simulink model "Modello_attuatore"  (R2023a)
settings: Solver=ode14x  StartTime=0.0  StopTime=3  FixedStep=dt_sim  RelTol=1e-3
values from neighbouring files (symbols this model uses):
  A1_la = 5.710000e-003    (= 0.00571)    [C1_Actuator_1_Data.m]
  A2_la = 5.710000e-003    (= 0.00571)    [C1_Actuator_1_Data.m]
  a_jetpipe_area = 0    [B2_Main_file_Double_Active_Standby_System.m]
  A_svfb = 79.12.*1E-9.*sqrt(pi)    [B2_Main_file_Double_Active_Standby_System.m]
  a_svfb0_1 = 1E-3    (= 0.001)    [B2_Main_file_Double_Active_Standby_System.m]
  a_svfb0_2 = 0    [B2_Main_file_Double_Active_Standby_System.m]
  Afl_sv = dfl_sv^2*pi/4    (= 2.01519637574e-09)    [C1_Actuator_1_Data.m]
  Ag_sv = 18e-6    (= 1.8e-05)    [C1_Actuator_1_Data.m]
  air_gap0_1 = 0    [B2_Main_file_Double_Active_Standby_System.m]
  air_gap_fault_time = 10000    [B2_Main_file_Double_Active_Standby_System.m]
  Asp_sv = 1.35e-5    (= 1.35e-05)    [C1_Actuator_1_Data.m]
  B0_sv = 0.460    (= 0.46)    [C1_Actuator_1_Data.m]
  b_airgap = 0.3    [B2_Main_file_Double_Active_Standby_System.m]
  b_fbspring = 2E-3    (= 0.002)    [B2_Main_file_Double_Active_Standby_System.m]
  b_max = 0*0.0001    (= 0)    [C1_Actuator_1_Data.m]
  beta = 800000000    [D4_Fluid.m]    (also in Rapporto_di_trasmissione.m = acos((L-t.*cos(alpha))./s))
  beta_LVDT = 0    [aggiunte.m]
  bf_sv = 0.45    [C1_Actuator_1_Data.m]
  bsp_sv = 0.25    [C1_Actuator_1_Data.m]
  C_svfb = 1    [B2_Main_file_Double_Active_Standby_System.m]
  Cdmax_sv = 0.7392    [C1_Actuator_1_Data.m]
  Cdmin_sv = 0.6428    [C1_Actuator_1_Data.m]
  CLa = 900000    [aggiunte.m]
  Csa_la = 0.02*sqrt(Ksa_la*Meq_la)    [C1_Actuator_1_Data.m]
  Del_on = 1    [B2_Main_file_Double_Active_Standby_System.m]
  demag0_1 = 0    [B2_Main_file_Double_Active_Standby_System.m]
  dfl_sv = 5.0654e-5    (= 5.0654e-05)    [C1_Actuator_1_Data.m]
  dt_sim = 1e-5    (= 1e-05)    [B2_Main_file_Double_Active_Standby_System.m]
  enable_jetpipe_distorsion = 0    [B2_Main_file_Double_Active_Standby_System.m]
  F_att_sv = 4    [C1_Actuator_1_Data.m]
  FH = FH+0.175*pi*Dd_se(ii)*(-0.884+0.0206*Hs_se(ii)-0.0001*(Hs_se(ii))^2)*Tw_se(ii)    [D2_Data_seal.m]
  first_cycle = 0    [B2_Main_file_Double_Active_Standby_System.m]
  flight_hours = 8    [B2_Main_file_Double_Active_Standby_System.m]
  g_sv = G_sv/l0_sv    (= 0)    [C1_Actuator_1_Data.m]
  Gamma_la = 1.667e4    (= 16670)    [C1_Actuator_1_Data.m]
  gap_ms = 0    [C1_Actuator_1_Data.m]
  Gq_sv = 0.069    [C1_Actuator_1_Data.m]
  Gust_stiffness_jetpipe = 1e8    (= 100000000)    [B2_Main_file_Double_Active_Standby_System.m]
  Gust_threshold = 10000    [B2_Main_file_Double_Active_Standby_System.m]
  h_fbspring = 1E-3    (= 0.001)    [B2_Main_file_Double_Active_Standby_System.m]
  h_sv = H_sv/l0_sv    (= 0)    [C1_Actuator_1_Data.m]
  hr_sv = 6e-6    (= 6e-06)    [C1_Actuator_1_Data.m]
  hyd_fluid_repl = 20    [B2_Main_file_Double_Active_Standby_System.m]
  imax_sv = 8e-3    (= 0.008)    [C1_Actuator_1_Data.m]
  Ja_sv = 1.0575e-5    (= 1.0575e-05)    [C1_Actuator_1_Data.m]
  jetpipe_initialpos = 0    [B2_Main_file_Double_Active_Standby_System.m]
  jetpipe_passage_area = 1    [B2_Main_file_Double_Active_Standby_System.m]
  k_airgap = 0.5/100*0.01    (= 5e-05)    [B2_Main_file_Double_Active_Standby_System.m]
  k_c0_jetpipe_area = 0*1e-1    (= 0)    [B2_Main_file_Double_Active_Standby_System.m]
  k_sv = mup_sv*Vp_sv/(2*B0_sv*l0_sv)-1    (= 16.0383594613)    [C1_Actuator_1_Data.m]
  Kf_sv = 301.6    [C1_Actuator_1_Data.m]
  KFPi = zeros(m,1)    [D2_Data_seal.m]
  Kli1 = 0    [C1_Actuator_1_Data.m]
  Kli2 = 0    [C1_Actuator_1_Data.m]
  Ksa_la = 12480000    [C1_Actuator_1_Data.m]
  Kw_sv = 14.5    [C1_Actuator_1_Data.m]
  l0_sv = 0.5e-3    (= 0.0005)    [C1_Actuator_1_Data.m]
  L_c = imax_sv    (= 0.008)    [C1_Actuator_1_Data.m]
  L_la1 = 0.059900    (= 0.0599)    [C1_Actuator_1_Data.m]
  L_la2 = 0.084800    (= 0.0848)    [C1_Actuator_1_Data.m]
  la_sv = 41e-3    (= 0.041)    [C1_Actuator_1_Data.m]
  lambda_LVDT = 0*0.005*1.5    (= 0)    [aggiunte.m]
  lf = 0.025    [C1_Actuator_1_Data.m]    (also in C2_Actuator_2_Data.m)
  LVDTsize0 = 1    [aggiunte.m]
  m_thermal = 0    [B2_Main_file_Double_Active_Standby_System.m]
  Mcyl_la = 30.425550    (= 30.42555)    [C1_Actuator_1_Data.m]
  Mrod_la = 11.313490    (= 11.31349)    [C1_Actuator_1_Data.m]
  msp_sv = 0.005    [C1_Actuator_1_Data.m]
  mua_sv = 4*pi/1e7    (= 1.25663706144e-06)    [C1_Actuator_1_Data.m]
  mup_sv = 1.1*4*pi/1e7    (= 1.38230076758e-06)    [C1_Actuator_1_Data.m]
  n1_sv = 1140    [C1_Actuator_1_Data.m]
  n2_sv = 1140    [C1_Actuator_1_Data.m]
  n_svfb = 3    [B2_Main_file_Double_Active_Standby_System.m]
  null_shift = -1+2*rand(1,1)    [B2_Main_file_Double_Active_Standby_System.m]
  null_shift_sign = -1+((-1+2*rand(1,1))>=0)*2    [B2_Main_file_Double_Active_Standby_System.m]
  OV_R1 = 0*2.344e-05    (= 0)    [C1_Actuator_1_Data.m]
  OV_R2 = 0*2.344e-05    (= 0)    [C1_Actuator_1_Data.m]
  OV_S1 = 0*2.344e-05    (= 0)    [C1_Actuator_1_Data.m]
  OV_S2 = 0*2.344e-05    (= 0)    [C1_Actuator_1_Data.m]
  P01_la = Pmean-DP_eq    [C1_Actuator_1_Data.m]
  P02_la = Pmean+DP_eq    [C1_Actuator_1_Data.m]
  perc_passage_area0_1 = 0    [B2_Main_file_Double_Active_Standby_System.m]
  Pocl_A = 0    [C1_Actuator_1_Data.m]
  Pocl_B = 0    [C1_Actuator_1_Data.m]
  Pr = 600000    [B2_Main_file_Double_Active_Standby_System.m]
  Ps = 35000000    [B2_Main_file_Double_Active_Standby_System.m]
  R_th1 = 0    [B2_Main_file_Double_Active_Standby_System.m]
  Remax_sv = 5000    [C1_Actuator_1_Data.m]
  Resistance = 1    [C1_Actuator_1_Data.m]
  rj_sv = 1e-6    (= 1e-06)    [C1_Actuator_1_Data.m]
  Rp02_svspring = 1014    [B2_Main_file_Double_Active_Standby_System.m]
  sigma_0LVDT = 0*0.01*1.5*5    (= 0)    [aggiunte.m]
  ST_AD = ceil(10000/fs_AD)/10000    [C1_Actuator_1_Data.m]
  sv_crackON1 = 0    [B2_Main_file_Double_Active_Standby_System.m]
  sv_crackON2 = 0    [B2_Main_file_Double_Active_Standby_System.m]
  T0 = 0    [aggiunte.m]
  tau_w1 = 0    [B2_Main_file_Double_Active_Standby_System.m]
  Temperature_threshold = 0    [B2_Main_file_Double_Active_Standby_System.m]
  V01_la = (Vm_la1+A1_la*(L_la1+x0_la))    (= 0.00040017393)    [C1_Actuator_1_Data.m]
  V02_la = (Vm_la2+A2_la*(L_la2-x0_la))    (= 0.00056652336)    [C1_Actuator_1_Data.m]
  Voltage_com = Resistance    (= 1)    [C1_Actuator_1_Data.m]
  Vp_sv = 5.67e3    (= 5670)    [C1_Actuator_1_Data.m]
  w_fb = 310    [C1_Actuator_1_Data.m]
  w_sv = W_sv/l0_sv    (= 0)    [C1_Actuator_1_Data.m]
  wsp_sv = 0.009334348785340    (= 0.00933434878534)    [C1_Actuator_1_Data.m]
  x0_la = 0    [C1_Actuator_1_Data.m]
  xf_sv_max = 3.05e-5    (= 3.05e-05)    [C1_Actuator_1_Data.m]
  xmax_sb = 5.5e-3    (= 0.0055)    [C1_Actuator_1_Data.m]
  xspmax_sv = 0.001250    (= 0.00125)    [C1_Actuator_1_Data.m]
  z_fb = 0.5    [C1_Actuator_1_Data.m]
undefined symbols (not defined in the file or in its folder): magnitude, Newton, R_sp_C, Raphson
libraries: simulink x13
(part 1 of 3)
settings Model: SimulationMode=accelerator  Creator=ciro1  LastModifiedBy=ciro1

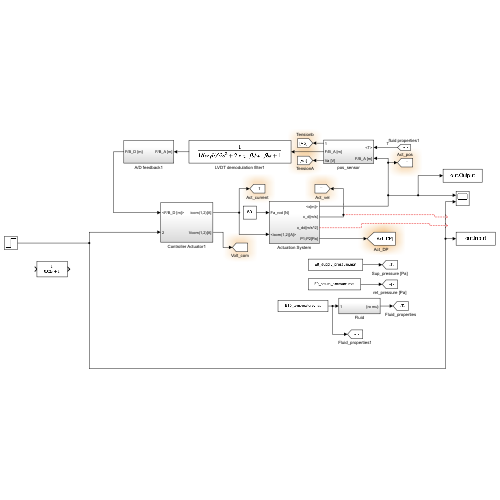
[thumbnail: Simulink's stored preview of the top-level diagram]
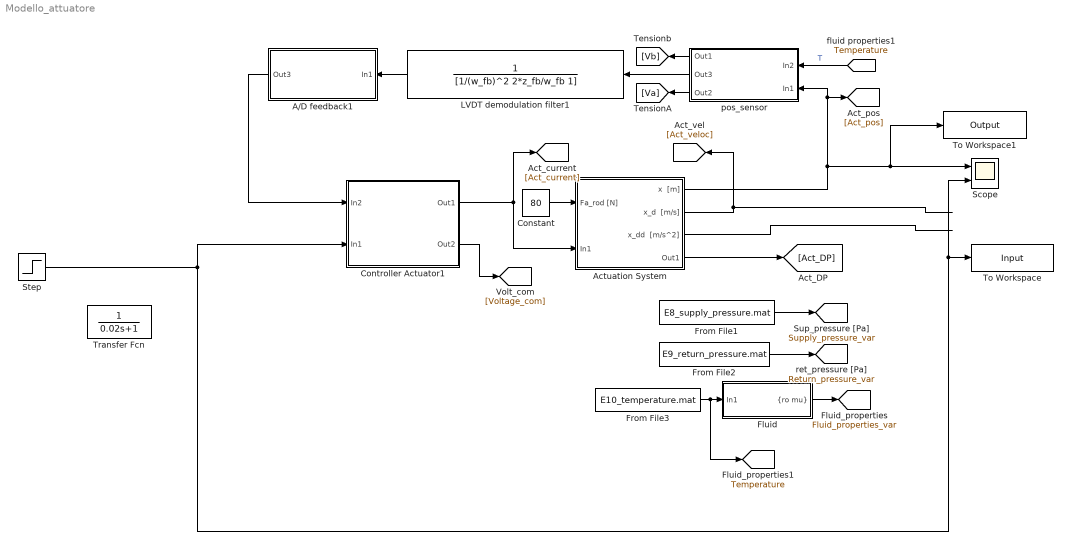
== system Modello_attuatore ==
  A/D feedback1 : Subsystem
  Actuation System : Subsystem
  Constant : Constant  Value=80
  Controller Actuator1 : Subsystem
  Fluid : Subsystem
  From File1 : FromFile  FileName=E8_supply_pressure.mat  SampleTime=dt_sim
  From File2 : FromFile  FileName=E9_return_pressure.mat  SampleTime=dt_sim
  From File3 : FromFile  FileName=E10_temperature.mat  SampleTime=dt_sim
  LVDT demodulation filter1 : TransferFcn  Denominator=[1/(w_fb)^2 2*z_fb/w_fb 1]
  Scope : Scope  NumInputPorts=2
  Step : Step  Time=0.1  After=0.02  SampleTime=0
  To Workspace : ToWorkspace  VariableName=Input  SampleTime=-1
  To Workspace1 : ToWorkspace  VariableName=Output  SampleTime=-1
  Transfer Fcn : TransferFcn  Denominator=[0.02 1]
  pos_sensor : Subsystem
  tag scope: Fluid_properties_var=global, Return_pressure_var=global, Supply_pressure_var=global, Temperature=global
  wires:
  pos_sensor/1(Out1) -> [Vb]
  pos_sensor/2(Out3) -> LVDT demodulation filter1/1
  A/D feedback1/1(Out3) -> Controller Actuator1/1(In2)
  Actuation System/3(x_dd  [m/s^2]) -> ?
  [Temperature] -> pos_sensor/1(In2)  "T"
  pos_sensor/3(Out2) -> [Va]
  Actuation System/2(x_d  [m/s]) -> [Act_veloc]
  Actuation System/4(Out1) -> [Act_DP]
  LVDT demodulation filter1/1 -> A/D feedback1/1(In1)
  Actuation System/1(x  [m]) -> To Workspace1/1, Scope/1, pos_sensor/2(In1), [Act_pos]
  Controller Actuator1/1(Out1) -> [Act_current], Actuation System/2(In1)
  Controller Actuator1/2(Out2) -> [Voltage_com]
  Fluid/1("{ro mu}") -> [Fluid_properties_var]
  From File2/1 -> [Return_pressure_var]
  From File3/1 -> [Temperature], Fluid/1(In1)
  From File1/1 -> [Supply_pressure_var]
  Step/1 -> Controller Actuator1/2(In1), Scope/2, To Workspace/1
  Constant/1 -> Actuation System/1(Fa_rod [N])

== system Modello_attuatore/A//D feedback1 ==
  In1 : Inport
  L_hight[ft]2 : Constant  Value=Del_on
  Product : Product  RndMeth=Zero
  Quantizer : Quantizer  QuantizationInterval=QI_AD
  Quantizer1 : Quantizer  QuantizationInterval=QI_AD
  "Sampler " : ZeroOrderHold  SampleTime=ST_AD
  Sum : Sum  Inputs=|++
  Uniform Random Number1 : UniformRandomNumber  Minimum=-4*2.5757e-006  Maximum=4*2.5757e-006  SampleTime=1
  Out3 : Outport
  wires:
  "Sampler "/1 -> Quantizer/1
  In1/1 -> "Sampler "/1  "F/B_A [m]"
  Uniform Random Number1/1 -> Quantizer1/1
  Quantizer/1 -> Sum/1  "F/B_D [m]"
  Sum/1 -> Out3/1  "F/B_D [m]"
  Product/1 -> Sum/2
  Quantizer1/1 -> Product/1  "Noise A/D"
  L_hight[ft]2/1 -> Product/2

== system Modello_attuatore/Actuation System ==
  Fa_rod [N] : Inport
  In1 : Inport  Port=2
  A2[m2]1 : Gain  Gain=60000
  Actuator : Subsystem
  Mux1 : Mux  Inputs=2
  Scope : Scope
  Servovalve : Subsystem
  imposed shutoff valve external position : Constant  Value=xmax_sb
  x  [m] : Outport
  x_d  [m/s] : Outport  Port=2
  x_dd  [m/s^2] : Outport  Port=3
  Out1 : Outport  Port=4
  wires:
  In1/1 -> Servovalve/2(In1)
  Actuator/2(Out3) -> x  [m]/1
  Actuator/3(Out1) -> x_d  [m/s]/1  "x_d[m/s]"
  Servovalve/1(Out4) -> Mux1/1, Actuator/1(In1)
  Servovalve/2(Out1) -> Actuator/2(In3), Mux1/2
  Actuator/1(Out2) -> Out1/1, Servovalve/1(In2)  "P1;P2[Pa]"
  imposed shutoff valve external position/1 -> Servovalve/3(In3)  "X_shutoff [m]"
  Mux1/1 -> A2[m2]1/1
  A2[m2]1/1 -> Scope/1
  Fa_rod [N]/1 -> Actuator/3(" ")
  Actuator/4(Out5) -> x_dd  [m/s^2]/1  "x_dd[m/s^2]"

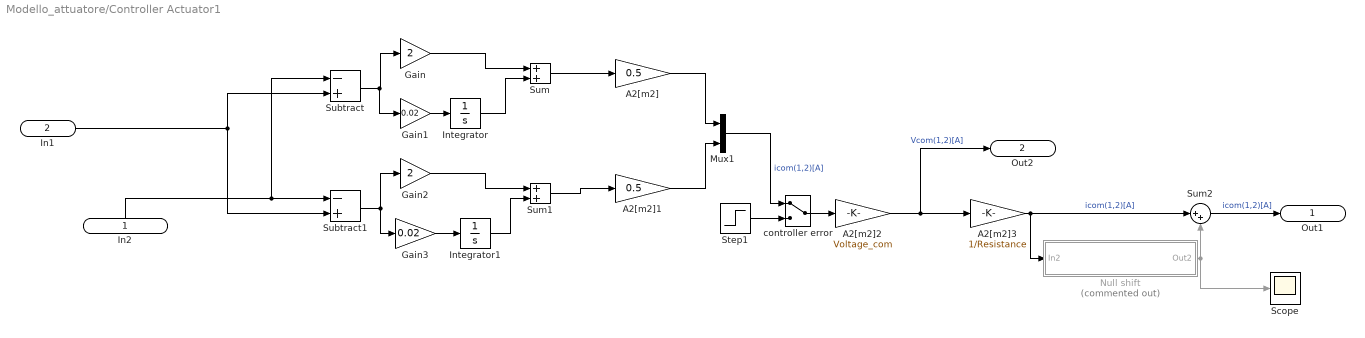
== system Modello_attuatore/Controller Actuator1 ==
  In2 : Inport
  In1 : Inport  Port=2
  A2[m2] : Gain  Gain=0.5
  A2[m2]1 : Gain  Gain=0.5
  A2[m2]2 : Gain  Gain=Voltage_com
  A2[m2]3 : Gain  Gain=1/Resistance
  Gain : Gain  Gain=2
  Gain1 : Gain  Gain=0.02
  Gain2 : Gain  Gain=2
  Gain3 : Gain  Gain=0.02
  Integrator : Integrator
  Integrator1 : Integrator
  Mux1 : Mux  Inputs=2
  Null shift : Subsystem  Commented=on
  Scope : Scope
  Step1 : Step  Time=0.3  After=L_c  SampleTime=0
  Subtract : Sum  Inputs=-+
  Subtract1 : Sum  Inputs=-+
  Sum : Sum
  Sum1 : Sum
  Sum2 : Sum  Inputs=|++
  controller error : ManualSwitch
  Out1 : Outport
  Out2 : Outport  Port=2
  wires:
  A2[m2]1/1 -> Mux1/2
  A2[m2]/1 -> Mux1/1
  In1/1 -> Subtract1/2, Subtract/2
  Mux1/1 -> controller error/1  "icom(1,2)[A]"
  controller error/1 -> A2[m2]2/1
  Step1/1 -> controller error/2
  A2[m2]2/1 -> A2[m2]3/1, Out2/1  "Vcom(1,2)[A]"
  A2[m2]3/1 -> Sum2/1, Null shift/1(In2)  "icom(1,2)[A]"
  Null shift/1(Out2) -> Sum2/2, Scope/1
  Sum2/1 -> Out1/1  "icom(1,2)[A]"
  Gain/1 -> Sum/1
  Subtract/1 -> Gain1/1, Gain/1
  Subtract1/1 -> Gain3/1, Gain2/1
  Gain2/1 -> Sum1/1
  Sum1/1 -> A2[m2]1/1
  Sum/1 -> A2[m2]/1
  In2/1 -> Subtract/1, Subtract1/1
  Gain1/1 -> Integrator/1
  Integrator/1 -> Sum/2
  Gain3/1 -> Integrator1/1
  Integrator1/1 -> Sum1/2

== system Modello_attuatore/Fluid ==
  In1 : Inport
  Mux2 : Mux  Inputs=2
  Product2 : Product  RndMeth=Zero
  tt : Fcn  Expr=(-0.85*u(1)+1015.4)*(1+20/8000)
  tt1 : Fcn  Expr=(1e-6*10^(0.3829*log10(u(1) +51)^4-1.8481*log10(u(1) +51)^3+2.2079*log10(u(1) +51)^2-1.1052*log10(u(1) +51)+2.9544))
  "{ro mu}" : Outport
  tag scope: only_viscosity_var=global
  wires:
  In1/1 -> tt1/1, tt/1
  tt/1 -> Mux2/1, Product2/1  "ro"
  Product2/1 -> Mux2/2, [only_viscosity_var]  "mu"
  tt1/1 -> Product2/2
  Mux2/1 -> "{ro mu}"/1

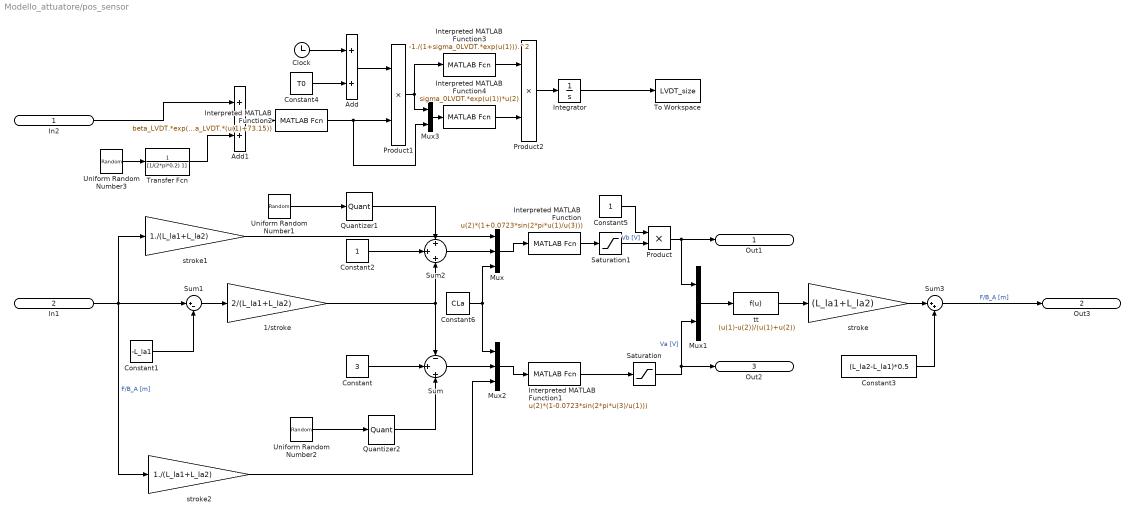
== system Modello_attuatore/pos_sensor ==
  In2 : Inport
  In1 : Inport  Port=2
  1/stroke : Gain  Gain=2/(L_la1+L_la2)  SaturateOnIntegerOverflow=on  OutDataTypeStr=Inherit: Same as input  ParamDataTypeStr=Inherit: Same as input
  Add : Sum
  Add1 : Sum
  Clock : Clock
  Constant : Constant  Value=3
  Constant1 : Constant  Value=-L_la1
  Constant2 : Constant
  Constant3 : Constant  Value=(L_la2-L_la1)*0.5
  Constant4 : Constant  Value=T0
  Constant5 : Constant
  Constant6 : Constant  Value=CLa
  Integrator : Integrator  InitialCondition=LVDTsize0
  Interpreted MATLAB Function : MATLABFcn  MATLABFcn=u(2)*(1+0.0723*sin(2*pi*u(1)/u(3)))
  Interpreted MATLAB Function1 : MATLABFcn  MATLABFcn=u(2)*(1-0.0723*sin(2*pi*u(3)/u(1)))
  Interpreted MATLAB Function2 : MATLABFcn  MATLABFcn=beta_LVDT.*exp(lambda_LVDT.*(u(1)+73.15))
  Interpreted MATLAB Function3 : MATLABFcn  MATLABFcn=-1./(1+sigma_0LVDT.*exp(u(1))).^2
  Interpreted MATLAB Function4 : MATLABFcn  MATLABFcn=sigma_0LVDT.*exp(u(1))*u(2)
  Mux : Mux  Inputs=3
  Mux1 : Mux  Inputs=2
  Mux2 : Mux  Inputs=3
  Mux3 : Mux  Inputs=2
  Product : Product
  Product1 : Product
  Product2 : Product
  Quantizer1 : Quantizer  QuantizationInterval=4/(2^14)
  Quantizer2 : Quantizer  QuantizationInterval=4/(2^14)
  Saturation : Saturate  UpperLimit=3  LowerLimit=1
  Saturation1 : Saturate  UpperLimit=3  LowerLimit=1
  Sum : Sum  Inputs=-|+|+
  Sum1 : Sum  Inputs=|+-
  Sum2 : Sum  Inputs=+|+|+
  Sum3 : Sum  Inputs=|++
  To Workspace : ToWorkspace  VariableName=LVDT_size  SaveFormat=Structure With Time  SampleTime=-1
  Transfer Fcn : TransferFcn  Denominator=[1/(2*pi*0.2) 1]
  Uniform Random Number1 : UniformRandomNumber  Minimum=-0.02*2  Maximum=0.02*2
  Uniform Random Number2 : UniformRandomNumber  Minimum=-0.02*2  Maximum=0.02*2
  Uniform Random Number3 : UniformRandomNumber  Minimum=-20  Maximum=20  Seed=rand(1)  SampleTime=10
  stroke : Gain  Gain=(L_la1+L_la2)  SaturateOnIntegerOverflow=on  OutDataTypeStr=Inherit: Same as input  ParamDataTypeStr=Inherit: Same as input
  stroke1 : Gain  Gain=1./(L_la1+L_la2)  SaturateOnIntegerOverflow=on  OutDataTypeStr=Inherit: Same as input  ParamDataTypeStr=Inherit: Same as input
  stroke2 : Gain  Gain=1./(L_la1+L_la2)  SaturateOnIntegerOverflow=on  OutDataTypeStr=Inherit: Same as input  ParamDataTypeStr=Inherit: Same as input
  tt : Fcn  Expr=(u(1)-u(2))/(u(1)+u(2))
  Out1 : Outport
  Out3 : Outport  Port=2
  Out2 : Outport  Port=3
  wires:
  In1/1 -> stroke2/1, stroke1/1, Sum1/1  "F/B_A [m]"
  Constant1/1 -> Sum1/2
  Sum1/1 -> 1/stroke/1
  Constant/1 -> Sum/2
  1/stroke/1 -> Sum/1, Sum2/3
  Constant2/1 -> Sum2/2
  Mux1/1 -> tt/1
  tt/1 -> stroke/1
  Sum3/1 -> Out3/1  "F/B_A [m]"
  Constant3/1 -> Sum3/2
  stroke/1 -> Sum3/1
  Uniform Random Number1/1 -> Quantizer1/1
  Uniform Random Number2/1 -> Quantizer2/1
  Quantizer1/1 -> Sum2/1
  Quantizer2/1 -> Sum/3
  Saturation/1 -> Out2/1, Mux1/2  "Va [V]"
  Sum2/1 -> Mux/2
  stroke1/1 -> Mux/1
  Interpreted MATLAB Function/1 -> Saturation1/1
  Mux/1 -> Interpreted MATLAB Function/1
  Mux2/1 -> Interpreted MATLAB Function1/1
  Interpreted MATLAB Function1/1 -> Saturation/1
  Product/1 -> Mux1/1, Out1/1
  Saturation1/1 -> Product/2  "Vb [V]"
  Constant4/1 -> Add/2
  Clock/1 -> Add/1
  Interpreted MATLAB Function2/1 -> Mux3/2, Product1/2
  Add/1 -> Product1/1
  Product1/1 -> Mux3/1, Interpreted MATLAB Function3/1
  Add1/1 -> Interpreted MATLAB Function2/1
  In2/1 -> Add1/1
  Uniform Random Number3/1 -> Transfer Fcn/1
  Transfer Fcn/1 -> Add1/2
  Interpreted MATLAB Function3/1 -> Product2/1
  Interpreted MATLAB Function4/1 -> Product2/2
  Product2/1 -> Integrator/1
  Integrator/1 -> To Workspace/1
  Mux3/1 -> Interpreted MATLAB Function4/1
  Constant5/1 -> Product/1
  stroke2/1 -> Mux2/3
  Sum/1 -> Mux2/2
  Constant6/1 -> Mux2/1, Mux/3

== system Modello_attuatore/Actuation System/Actuator ==
  In1 : Inport
  In3 : Inport  Port=2
  " " : Inport  Port=3
  Add1 : Sum  Inputs=+|-
  Add2 : Sum  Inputs=+|-
  Add3 : Sum  Inputs=+|-
  Chamber equation : Subsystem
  Constant : Constant  Value=beta
  Rod : Subsystem
  Sleeve : Subsystem
  Out2 : Outport
  Out3 : Outport  Port=2
  Out1 : Outport  Port=3
  Out5 : Outport  Port=4
  wires:
  Chamber equation/1(Out3) -> Out2/1, Rod/3(In2), Sleeve/2(In2)  "P1;P2[Pa]"
  Constant/1 -> Chamber equation/3(In2)  "beta[Pa]"
  In1/1 -> Chamber equation/1(In4)
  In3/1 -> Chamber equation/2(In1)
  " "/1 -> Rod/2(In6)  "Fa_rod [N]"
  Sleeve/1(Out4) -> Add1/2  "xC[m]"
  Rod/3(Out4) -> Add1/1  "xR[m]"
  Rod/2(Out3) -> Add2/1  "xR_d[m/s]"
  Sleeve/2(Out3) -> Add2/2  "xC_d[m/s]"
  Add2/1 -> [x_d], Out1/1  "x_d[m/s]"
  Add1/1 -> Out3/1, [x]  "x[m]"
  [x_d] -> Chamber equation/4(In3)  "x_d[m/s]"
  [x] -> Chamber equation/5(In5)  "x[m]"
  Rod/4(Out2) -> Sleeve/1(In4)
  [x_d] -> Rod/1(In1)  "x_d[m/s]"
  Add3/1 -> Out5/1  "x_dd[m/s^2]"
  Rod/1(Out1) -> Add3/1
  Sleeve/3(Out1) -> Add3/2

== system Modello_attuatore/Actuation System/Servovalve ==
  In2 : Inport
  In1 : Inport  Port=2
  In3 : Inport  Port=3
  Demux : Demux  Outputs=2
  Servovalve Dynamic : Subsystem
  Spool : Subsystem
  Terminator : Terminator
  Terminator1 : Terminator
  Terminator2 : Terminator
  Out4 : Outport
  Out1 : Outport  Port=2
  tag scope: Act_spool=global
  wires:
  In1/1 -> Servovalve Dynamic/3(In4)  "icom1;2[A]"
  Servovalve Dynamic/1(Out1) -> Spool/3(In4), [Act_spool]  "xs[m]"
  [Fluid_properties_var] -> Servovalve Dynamic/4(In3), Spool/4(In6)  "ro;mu"
  Servovalve Dynamic/2(Out2) -> Terminator2/1
  [Supply_pressure_var] -> Servovalve Dynamic/1(In1), Spool/1(In1)  "Ps[Pa]"
  [Return_pressure_var] -> Spool/2(In5), Servovalve Dynamic/2(In2)  "Pr[Pa]"
  Spool/3(Out1) -> Out4/1  "Q1[m3/s]"
  Spool/4(Out3) -> Out1/1  "Q2[m3/s]"
  Spool/1(Out2) -> Terminator/1  "Qsup[m3/s]"
  Spool/2(Out4) -> Terminator1/1  "Qret[m3/s]"
  In2/1 -> Demux/1
  Demux/1 -> Spool/5(In2)  "P1_sb[Pa]"
  Demux/2 -> Spool/6(In3)  "P2_sb[Pa]"
  In3/1 -> Spool/7(In7)

== system Modello_attuatore/Controller Actuator1/Null shift ==
  In2 : Inport
  A2[m2]1 : Gain  Gain=5/300
  A2[m2]4 : Gain  Gain=3/500
  Abs1 : Abs  SaturateOnIntegerOverflow=off
  Abs2 : Abs  SaturateOnIntegerOverflow=off
  Add1 : Sum  Inputs=+|-
  Add2 : Sum  Inputs=+|+
  Add3 : Sum  Inputs=+|-
  Constant1 : Constant  Value=Pr
  Constant2 : Constant  Value=null_shift_sign
  Constant3 : Constant  Value=20
  Constant4 : Constant  Value=null_shift
  From File2 : FromFile  FileName=E9_return_pressure.mat  SampleTime=dt_sim
  From File3 : FromFile  FileName=E10_temperature.mat  SampleTime=dt_sim
  Product1 : Product  Inputs=**/*  SaturateOnIntegerOverflow=on  OutDataTypeStr=Inherit: Same as first input
  Product2 : Product  Inputs=**/*  SaturateOnIntegerOverflow=on  OutDataTypeStr=Inherit: Same as first input
  Out2 : Outport
  wires:
  From File2/1 -> Add3/1
  Constant1/1 -> Add3/2, Product1/3
  Add3/1 -> Product1/2
  Constant2/1 -> Product1/4
  Product1/1 -> A2[m2]4/1
  In2/1 -> Abs2/1
  From File3/1 -> Add1/1
  Constant3/1 -> Add1/2, Product2/3
  Add1/1 -> Abs1/1
  Constant4/1 -> Product2/4
  Abs1/1 -> Product2/2
  Product2/1 -> A2[m2]1/1
  A2[m2]1/1 -> Add2/2
  A2[m2]4/1 -> Add2/1
  Add2/1 -> Out2/1  "Current shift [A]"
  Abs2/1 -> Product1/1, Product2/1

== system Modello_attuatore/Actuation System/Actuator/Chamber equation ==
  note: Q2_fb[m3/s]
  In4 : Inport
  In1 : Inport  Port=2
  In2 : Inport  Port=3
  In3 : Inport  Port=4
  In5 : Inport  Port=5
  Add : Sum  Inputs=+|-
  Chamber 1 : Subsystem
  Chamber 2 : Subsystem
  External leakage 1 : Fcn  Expr=Kli1*u(1)+Kli2*sqrt(abs(u(1)))
  External leakage 2 : Fcn  Expr=Kli1*u(1)+Kli2*sqrt(abs(u(1)))
  Internal leakage : Subsystem
  Mux : Mux  Inputs=2
  Out3 : Outport
  wires:
  In4/1 -> Chamber 1/1(In1)  "Q1_fb[m3/s]"
  External leakage 1/1 -> Chamber 1/6(In2)  "Qle1[m3/s]"
  Internal leakage/1(Out1) -> Chamber 1/5(In3), Chamber 2/2(In3)  "Qli[m3/s]"
  Add/1 -> Internal leakage/1(In6)  "DP[Pa]"
  Chamber 1/1(Out1) -> External leakage 1/1, Add/1, Mux/1  "P1[Pa]"
  Chamber 2/1(Out1) -> External leakage 2/1, Add/2, Mux/2  "P2[Pa]"
  In2/1 -> Chamber 1/2(In6), Chamber 2/5(In6)  "beta[Pa]"
  In3/1 -> Chamber 1/3(In5), Chamber 2/4(In5)  "x_d[m/s]"
  In5/1 -> Chamber 1/4(In4), Chamber 2/3(In4)  "x[m]"
  Mux/1 -> Out3/1  "P1;P2[Pa]"
  In1/1 -> Chamber 2/6(In1)
  External leakage 2/1 -> Chamber 2/1(In2)  "Qle2[m3/s]"

== system Modello_attuatore/Actuation System/Actuator/Rod ==
  In1 : Inport
  In6 : Inport  Port=2
  In2 : Inport  Port=3
  1/Mrod[1/kg] : Gain  Gain=1/(Mrod_la+27.5)
  A1[m2] : Gain  Gain=A1_la
  A2[m2] : Gain  Gain=A2_la
  Add1 : Sum  Inputs=+|-|+
  Demux : Demux  Outputs=2
  Double Integrator : Subsystem
  Friction1 : Subsystem
  Gamma[Ns/m] : Gain  Gain=Gamma_la
  Out1 : Outport
  Out3 : Outport  Port=2
  Out4 : Outport  Port=3
  Out2 : Outport  Port=4
  wires:
  Add1/1 -> Friction1/2(In1)  "Fact[N]"
  Demux/1 -> A1[m2]/1  "P1[Pa]"
  Demux/2 -> A2[m2]/1  "P2[Pa]"
  In2/1 -> Demux/1, Friction1/1(In3)  "P1;P2[Pa]"
  Friction1/2(Out1) -> 1/Mrod[1/kg]/1
  1/Mrod[1/kg]/1 -> Out1/1, Double Integrator/1(In1)  "xR_dd[m2/s]"
  Double Integrator/2(Out2) -> Out3/1, Friction1/4(In2)  "xR_d[m/s]"
  A1[m2]/1 -> Add1/1
  A2[m2]/1 -> Add1/2
  Double Integrator/1(Out1) -> Out4/1  "xR[m]"
  In1/1 -> Gamma[Ns/m]/1  "x_d[m/s]"
  Friction1/1(Out2) -> Out2/1  "Ffrict[N]"
  Friction1/3(Out3) -> Double Integrator/2(In2)
  Double Integrator/3(Out3) -> Friction1/5(In4)
  In6/1 -> Add1/3  "Fext[N]"
  Gamma[Ns/m]/1 -> Friction1/3(In5)

== system Modello_attuatore/Actuation System/Actuator/Sleeve ==
  In4 : Inport
  In2 : Inport  Port=2
  1/Mcyl[1/kg] : Gain  Gain=1/Mcyl_la
  A1[m2] : Gain  Gain=A1_la
  A2[m2] : Gain  Gain=A2_la
  Add1 : Sum  Inputs=-|+|-
  Add3 : Sum  Inputs=+|-
  Backlash : Subsystem
  Demux : Demux  Outputs=2
  Integrator : Integrator
  Integrator1 : Integrator
  Out4 : Outport
  Out3 : Outport  Port=2
  Out1 : Outport  Port=3
  wires:
  Demux/1 -> A1[m2]/1  "P1[Pa]"
  Demux/2 -> A2[m2]/1  "P2[Pa]"
  In2/1 -> Demux/1  "P1;P2[Pa]"
  A1[m2]/1 -> Add1/1
  A2[m2]/1 -> Add1/2
  Integrator/1 -> Integrator1/1, Out3/1, Backlash/1(In2)  "xC_d[m/s]"
  Integrator1/1 -> Out4/1, Backlash/2(In1)  "xC [m]"
  In4/1 -> Add1/3  "Ffrict[N]"
  1/Mcyl[1/kg]/1 -> Out1/1, Integrator/1  "xC_dd [m/s^2]"
  Add1/1 -> Add3/1  "Fact[N]"
  Backlash/1(Out1) -> Add3/2  "Fext_sl[N]"
  Add3/1 -> 1/Mcyl[1/kg]/1

== system Modello_attuatore/Actuation System/Servovalve/Servovalve Dynamic ==
  In1 : Inport
  In2 : Inport  Port=2
  In4 : Inport  Port=3
  In3 : Inport  Port=4
  Crack propagation : Subsystem
  First Stage Leakage : Subsystem
  Hydraulic amplifier : Subsystem
  Jet pipe dynamic : Subsystem
  Saturation2 : Saturate  UpperLimit=Ps-Pr  LowerLimit=-(Ps-Pr)
  Spool  dynamic : Subsystem
  Torque Motor : Subsystem
  Out1 : Outport
  Out2 : Outport  Port=2
  wires:
  In4/1 -> Torque Motor/1(In4)  "icom(1;2)[A]"
  In2/1 -> First Stage Leakage/2(In2), Hydraulic amplifier/3(In3)  "Pr[Pa]"
  In1/1 -> First Stage Leakage/1(In1), Hydraulic amplifier/2(In2)  "Ps[Pa]"
  First Stage Leakage/1(Out1) -> Out2/1  "QLfs[m3/s]"
  In3/1 -> First Stage Leakage/3(In4)  "ro;mu"
  Spool  dynamic/2(Out2) -> Hydraulic amplifier/4(In1)  "dxs[m/s]"
  Spool  dynamic/1(Out1) -> Jet pipe dynamic/1(In1), Out1/1  "xs[m]"
  Hydraulic amplifier/1(Out1) -> Saturation2/1  "dP[Pa]"
  Jet pipe dynamic/1(Out1) -> Spool  dynamic/1(In1), Hydraulic amplifier/1(In4)  "xf[m]"
  Saturation2/1 -> Spool  dynamic/2(In4)
  Jet pipe dynamic/2(Out2) -> Torque Motor/2(In1)
  Torque Motor/1(Out1) -> Crack propagation/1(Tb [N/m]), Jet pipe dynamic/2(In4)  "Torque [Nm]"
  Crack propagation/1(Kw_mod) -> Jet pipe dynamic/3(In2), Spool  dynamic/3(In2)
  [flight_time] -> Hydraulic amplifier/5(In5)

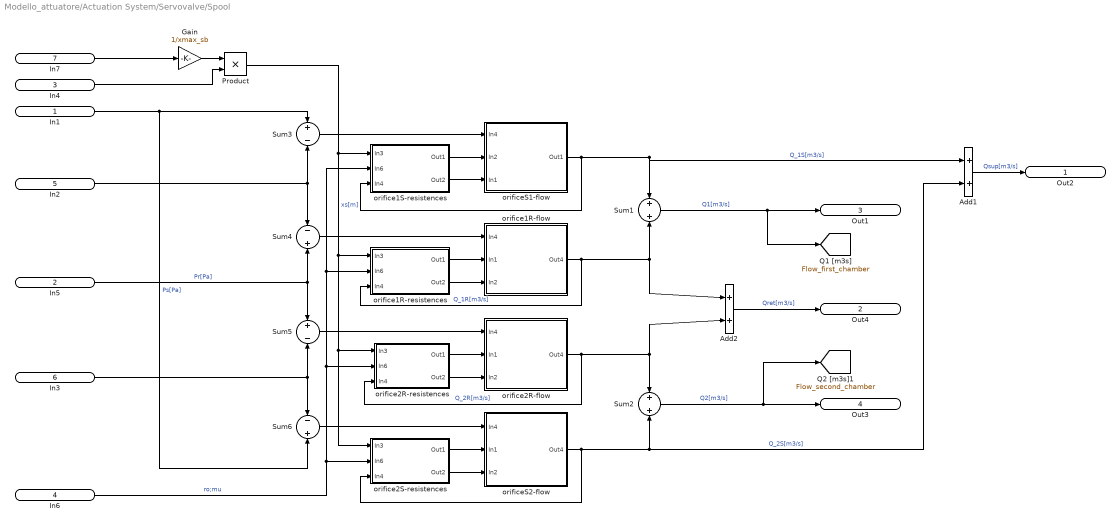
== system Modello_attuatore/Actuation System/Servovalve/Spool ==
  In1 : Inport
  In5 : Inport  Port=2
  In4 : Inport  Port=3
  In6 : Inport  Port=4
  In2 : Inport  Port=5
  In3 : Inport  Port=6
  In7 : Inport  Port=7
  Add1 : Sum  Inputs=+|+
  Add2 : Sum  Inputs=+|+
  Gain : Gain  Gain=1/xmax_sb
  Product : Product  RndMeth=Zero
  Sum1 : Sum  Inputs=+|+  SaturateOnIntegerOverflow=on
  Sum2 : Sum  Inputs=+|+  SaturateOnIntegerOverflow=on
  Sum3 : Sum  Inputs=+-  SaturateOnIntegerOverflow=on
  Sum4 : Sum  Inputs=-|+  SaturateOnIntegerOverflow=on
  Sum5 : Sum  Inputs=+|-  SaturateOnIntegerOverflow=on
  Sum6 : Sum  Inputs=-+  SaturateOnIntegerOverflow=on
  orifice1R-flow : Subsystem
  orifice1R-resistences : Subsystem
  orifice1S-resistences : Subsystem
  orifice2R-flow : Subsystem
  orifice2R-resistences : Subsystem
  orifice2S-resistences : Subsystem
  orificeS1-flow : Subsystem
  orificeS2-flow : Subsystem
  Out2 : Outport
  Out4 : Outport  Port=2
  Out1 : Outport  Port=3
  Out3 : Outport  Port=4
  tag scope: Flow_first_chamber=global, Flow_second_chamber=global
  wires:
  orificeS1-flow/1(Out1) -> Sum1/1, Add1/1, orifice1S-resistences/3(In4)  "Q_1S[m3/s]"
  orifice1R-flow/1(Out4) -> Add2/1, Sum1/2, orifice1R-resistences/3(In4)  "Q_1R[m3/s]"
  Sum4/1 -> orifice1R-flow/1(In4)
  Sum3/1 -> orificeS1-flow/1(In4)
  In2/1 -> Sum4/1, Sum3/2
  In3/1 -> Sum5/2, Sum6/1
  In1/1 -> Sum6/2, Sum3/1  "Ps[Pa]"
  Sum1/1 -> Out1/1, [Flow_first_chamber]  "Q1[m3/s]"
  Sum2/1 -> Out3/1, [Flow_second_chamber]  "Q2[m3/s]"
  orifice2S-resistences/1(Out1) -> orificeS2-flow/2(In1)
  Sum5/1 -> orifice2R-flow/1(In4)
  orifice2R-flow/1(Out4) -> Add2/2, Sum2/1, orifice2R-resistences/3(In4)  "Q_2R[m3/s]"
  orifice2S-resistences/2(Out2) -> orificeS2-flow/3(In2)
  orificeS2-flow/1(Out4) -> Sum2/2, Add1/2, orifice2S-resistences/3(In4)  "Q_2S[m3/s]"
  In5/1 -> Sum5/1, Sum4/2  "Pr[Pa]"
  Add1/1 -> Out2/1  "Qsup[m3/s]"
  Add2/1 -> Out4/1  "Qret[m3/s]"
  Product/1 -> orifice1S-resistences/1(In3), orifice2R-resistences/1(In3), orifice2S-resistences/1(In3), orifice1R-resistences/1(In3)  "xs[m]"
  In6/1 -> orifice1S-resistences/2(In6), orifice1R-resistences/2(In6), orifice2R-resistences/2(In6), orifice2S-resistences/2(In6)  "ro;mu"
  orifice2R-resistences/1(Out1) -> orifice2R-flow/2(In1)
  orifice2R-resistences/2(Out2) -> orifice2R-flow/3(In2)
  Sum6/1 -> orificeS2-flow/1(In4)
  orifice1R-resistences/1(Out1) -> orifice1R-flow/2(In1)
  orifice1R-resistences/2(Out2) -> orifice1R-flow/3(In2)
  orifice1S-resistences/1(Out1) -> orificeS1-flow/2(In2)
  orifice1S-resistences/2(Out2) -> orificeS1-flow/3(In1)
  In7/1 -> Gain/1
  Gain/1 -> Product/1
  In4/1 -> Product/2

== system Modello_attuatore/Actuation System/Actuator/Chamber equation/Chamber 1 ==
  In1 : Inport
  In6 : Inport  Port=2
  In5 : Inport  Port=3
  In4 : Inport  Port=4
  In3 : Inport  Port=5
  In2 : Inport  Port=6
  Integrator : Integrator  InitialCondition=P01_la  LimitOutput=on  UpperSaturationLimit=Ps  LowerSaturationLimit=Pr
  Mux : Mux  Inputs=6
  chamber1 equation : Fcn  Expr=u(2)*(u(1)-u(6)-u(5)-u(3)*A1_la)/(V01_la+u(4)*A1_la)
  Out1 : Outport
  wires:
  In1/1 -> Mux/1  "Q1[m3/s]"
  In2/1 -> Mux/6  "Qle1[m3/s]"
  In3/1 -> Mux/5  "Qli[m3/s]"
  In4/1 -> Mux/4  "z[m]"
  In5/1 -> Mux/3  "z_d[m/s]"
  In6/1 -> Mux/2  "beta[Pa]"
  chamber1 equation/1 -> Integrator/1  "dP1[Pa/s]"
  Integrator/1 -> Out1/1  "P1[Pa]"
  Mux/1 -> chamber1 equation/1

== system Modello_attuatore/Actuation System/Actuator/Chamber equation/Chamber 2 ==
  In2 : Inport
  In3 : Inport  Port=2
  In4 : Inport  Port=3
  In5 : Inport  Port=4
  In6 : Inport  Port=5
  In1 : Inport  Port=6
  Integrator : Integrator  InitialCondition=P02_la  LimitOutput=on  UpperSaturationLimit=Ps  LowerSaturationLimit=Pr
  Mux : Mux  Inputs=6
  chamber2 equation : Fcn  Expr=u(2)*(u(1)-u(6)+u(5)+u(3)*A2_la)/(V02_la-u(4)*A2_la)
  Out1 : Outport
  wires:
  In1/1 -> Mux/1  "Q2[m3/s]"
  Mux/1 -> chamber2 equation/1
  In2/1 -> Mux/6  "Qle2[m3/s]"
  In3/1 -> Mux/5  "Qli[m3/s]"
  In4/1 -> Mux/4  "z[m]"
  In5/1 -> Mux/3  "z_d[m/s]"
  In6/1 -> Mux/2  "beta[Pa]"
  chamber2 equation/1 -> Integrator/1  "dP2[Pa/s]"
  Integrator/1 -> Out1/1  "P2[Pa]"

== system Modello_attuatore/Actuation System/Actuator/Chamber equation/Internal leakage ==
  In6 : Inport
  Internal leakage : Fcn  Expr=Kli1*u(1)+Kli2*sqrt(abs(u(1)))*u(2)
  Mux : Mux  Inputs=2
  Sign : Signum
  Out1 : Outport
  wires:
  In6/1 -> Sign/1, Mux/1  "DP[Pa]"
  Sign/1 -> Mux/2
  Mux/1 -> Internal leakage/1
  Internal leakage/1 -> Out1/1  "Qli[m3/s]"

== system Modello_attuatore/Actuation System/Actuator/Rod/Double Integrator ==
  In1 : Inport
  In2 : Inport  Port=2
  Abs : Abs  SaturateOnIntegerOverflow=off
  Compare To Constant : simulink/Logic and Bit Operations/Compare To Constant  relop===  const=1  OutDataTypeStr=boolean
  Compare To Constant1 : simulink/Logic and Bit Operations/Compare To Constant  relop===  const=1  OutDataTypeStr=boolean
  Integrator : Integrator  ExternalReset=rising  ShowStatePort=on
  Integrator1 : Integrator  InitialCondition=x0_la  LimitOutput=on  UpperSaturationLimit=L_la2  LowerSaturationLimit=-L_la1  ShowSaturationPort=on
  Limit : Subsystem
  Logical Operator : Logic  Operator=OR  AllPortsSameDT=off  OutDataTypeStr=boolean
  Out1 : Outport
  Out2 : Outport  Port=2
  Out3 : Outport  Port=3
  wires:
  Integrator/1 -> Integrator1/1, Out2/1  "xR_d[m/s]"
  Integrator1/1 -> Out1/1  "xR[m]"
  Limit/1(Out2) -> Integrator/1
  Integrator1/2 -> Limit/2(In1), Abs/1  "limit xatt"
  In1/1 -> Limit/1(In2)  "xR_dd[m/s2]"
  Abs/1 -> Compare To Constant/1
  In2/1 -> Compare To Constant1/1
  Compare To Constant1/1 -> Logical Operator/1
  Compare To Constant/1 -> Logical Operator/2
  Logical Operator/1 -> Integrator/2
  Integrator/State -> Out3/1  "zero-crossing"

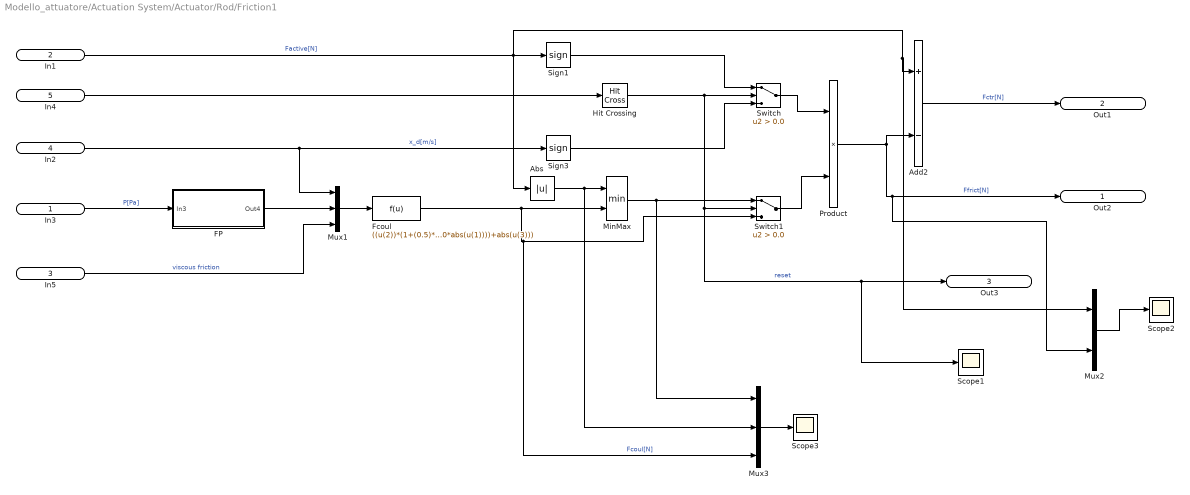
== system Modello_attuatore/Actuation System/Actuator/Rod/Friction1 ==
  In3 : Inport
  In1 : Inport  Port=2
  In5 : Inport  Port=3
  In2 : Inport  Port=4
  In4 : Inport  Port=5
  Abs : Abs  SaturateOnIntegerOverflow=off
  Add2 : Sum  Inputs=+|-
  FP : Subsystem
  Fcoul : Fcn  Expr=((u(2))*(1+(0.5)*exp(-10*abs(u(1))))+abs(u(3)))
  Hit Crossing : HitCross  HitCrossingOffset=0.0
  MinMax : MinMax  Inputs=2
  Mux1 : Mux  Inputs=3
  Mux2 : Mux  Inputs=2
  Mux3 : Mux  Inputs=3
  Product : Product  RndMeth=Zero
  Scope1 : Scope
  Scope2 : Scope
  Scope3 : Scope
  Sign1 : Signum
  Sign3 : Signum
  Switch : Switch  Criteria=u2 > Threshold  Threshold=0.0  SaturateOnIntegerOverflow=off  InputSameDT=off
  Switch1 : Switch  Criteria=u2 > Threshold  Threshold=0.0  SaturateOnIntegerOverflow=off  InputSameDT=off
  Out2 : Outport
  Out1 : Outport  Port=2
  Out3 : Outport  Port=3
  wires:
  Fcoul/1 -> MinMax/2, Mux3/3, Switch1/3  "Fcoul[N]"
  FP/1(Out4) -> Mux1/2
  In3/1 -> FP/1(In3)  "P[Pa]"
  Mux1/1 -> Fcoul/1
  In2/1 -> Mux1/1, Sign3/1  "x_d[m/s]"
  Add2/1 -> Out1/1  "Fctr[N]"
  Abs/1 -> Mux3/2, MinMax/1
  In1/1 -> Sign1/1, Abs/1, Mux2/1, Add2/1  "Factive[N]"
  Hit Crossing/1 -> Switch1/2, Scope1/1, Out3/1, Switch/2  "reset"
  Sign1/1 -> Switch/1
  Switch/1 -> Product/1
  MinMax/1 -> Mux3/1, Switch1/1
  Product/1 -> Add2/2, Mux2/2, Out2/1  "Ffrict[N]"
  In4/1 -> Hit Crossing/1
  Switch1/1 -> Product/2
  Sign3/1 -> Switch/3
  In5/1 -> Mux1/3  "viscous friction"
  Mux2/1 -> Scope2/1
  Mux3/1 -> Scope3/1

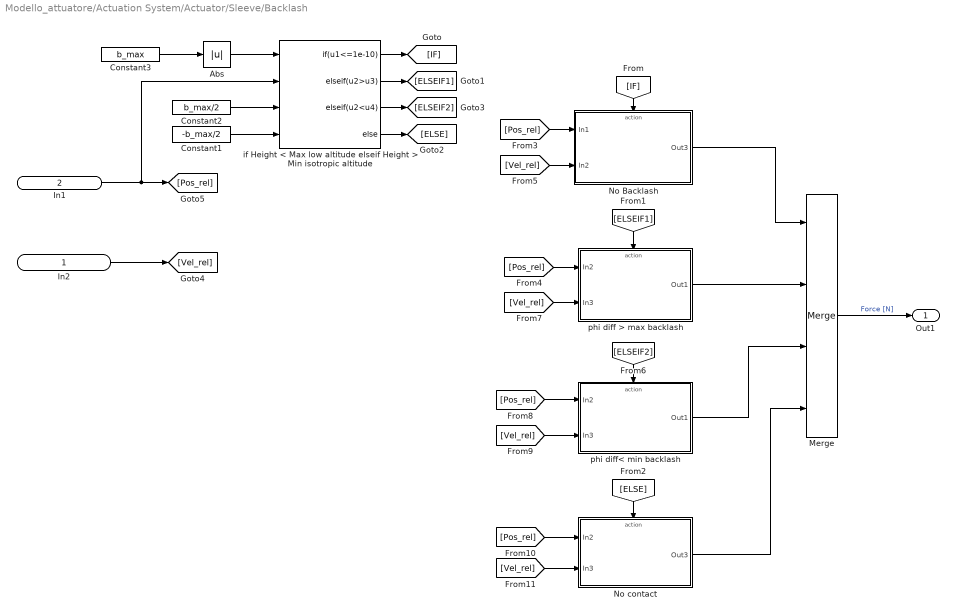
== system Modello_attuatore/Actuation System/Actuator/Sleeve/Backlash ==
  In2 : Inport
  In1 : Inport  Port=2
  Abs : Abs  SaturateOnIntegerOverflow=off
  Constant1 : Constant  Value=-b_max/2
  Constant2 : Constant  Value=b_max/2
  Constant3 : Constant  Value=b_max
  Merge : Merge  Inputs=4
  No Backlash : Subsystem  TreatAsAtomicUnit=on
  No contact : Subsystem  TreatAsAtomicUnit=on
  "if Height < Max low altitude elseif Height > Min isotropic altitude " : If  NumInputs=4  IfExpression=u1<=1e-10  ElseIfExpressions=u2>u3, u2<u4
  phi diff > max backlash : Subsystem  TreatAsAtomicUnit=on
  phi diff< min backlash : Subsystem  TreatAsAtomicUnit=on
  Out1 : Outport
  wires:
  "if Height < Max low altitude elseif Height > Min isotropic altitude "/1 -> [IF]
  "if Height < Max low altitude elseif Height > Min isotropic altitude "/2 -> [ELSEIF1]
  "if Height < Max low altitude elseif Height > Min isotropic altitude "/4 -> [ELSE]
  Abs/1 -> "if Height < Max low altitude elseif Height > Min isotropic altitude "/1
  In1/1 -> [Pos_rel], "if Height < Max low altitude elseif Height > Min isotropic altitude "/2
  Constant2/1 -> "if Height < Max low altitude elseif Height > Min isotropic altitude "/3
  Constant1/1 -> "if Height < Max low altitude elseif Height > Min isotropic altitude "/4
  "if Height < Max low altitude elseif Height > Min isotropic altitude "/3 -> [ELSEIF2]
  In2/1 -> [Vel_rel]
  [Pos_rel] -> No Backlash/1(In1)
  [Vel_rel] -> No Backlash/2(In2)
  [ELSEIF1] -> phi diff > max backlash/Action
  [IF] -> No Backlash/Action
  [Vel_rel] -> phi diff > max backlash/2(In3)
  [Pos_rel] -> phi diff > max backlash/1(In2)
  [ELSEIF2] -> phi diff< min backlash/Action
  [Vel_rel] -> phi diff< min backlash/2(In3)
  [Pos_rel] -> phi diff< min backlash/1(In2)
  No Backlash/1(Out3) -> Merge/1
  phi diff > max backlash/1(Out1) -> Merge/2
  phi diff< min backlash/1(Out1) -> Merge/3
  Merge/1 -> Out1/1  "Force [N]"
  [ELSE] -> No contact/Action
  No contact/1(Out3) -> Merge/4
  [Pos_rel] -> No contact/1(In2)
  [Vel_rel] -> No contact/2(In3)
  Constant3/1 -> Abs/1

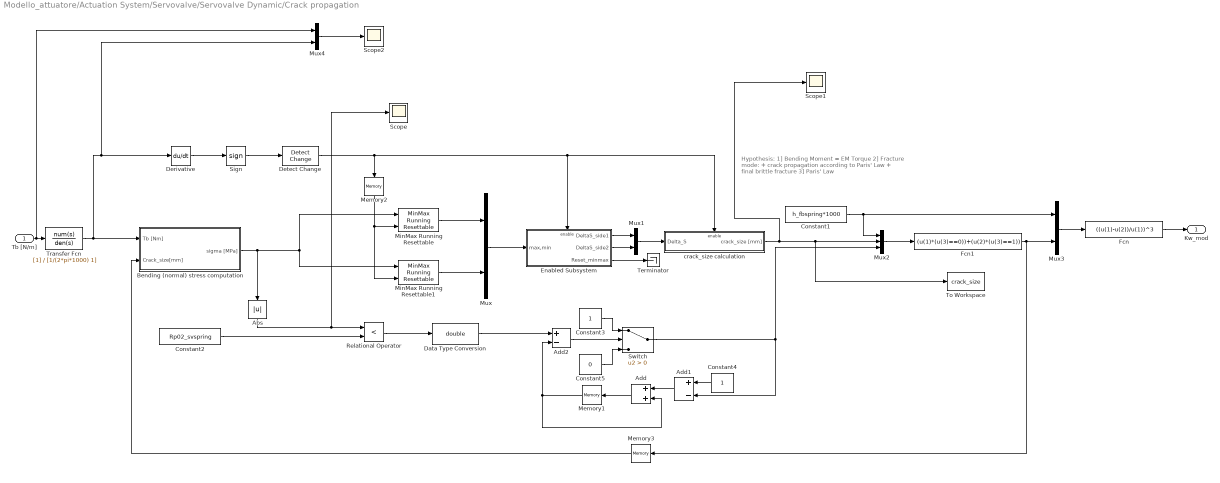
== system Modello_attuatore/Actuation System/Servovalve/Servovalve Dynamic/Crack propagation ==
  note: Hypothesis:
      | 1] Bending Moment = EM Torque
      | 2] Fracture mode:
      | 		+ crack propagation according to Paris' Law
      | 		+ final brittle fracture
      | 3] Paris' Law
  Tb [N/m] : Inport
  Abs : Abs  SaturateOnIntegerOverflow=off
  Add : Sum
  Add1 : Sum  Inputs=+-
  Add2 : Sum  Inputs=+-
  Bending (normal) stress computation : Subsystem
  Constant1 : Constant  Value=h_fbspring*1000
  Constant2 : Constant  Value=Rp02_svspring
  Constant3 : Constant
  Constant4 : Constant
  Constant5 : Constant  Value=0
  Data Type Conversion : DataTypeConversion  OutDataTypeStr=double  SaturateOnIntegerOverflow=off  RndMeth=Floor
  Derivative : Derivative
  Detect Change : simulink/Logic and Bit Operations/Detect Change  vinit=0  OutDataTypeStr=uint8
  Enabled Subsystem : Subsystem  TreatAsAtomicUnit=on
  Fcn : Fcn  Expr=((u(1)-u(2))/u(1))^3
  Fcn1 : Fcn  Expr=(u(1)*(u(3)==0))+(u(2)*(u(3)==1))
  Memory1 : Memory
  Memory2 : Memory
  Memory3 : Memory
  MinMax Running Resettable : simulink/Math Operations/MinMax Running Resettable  Function=max  vinit=0.0
  MinMax Running Resettable1 : simulink/Math Operations/MinMax Running Resettable  Function=min  vinit=0.0
  Mux{,1,3..4} (4 alike) : Mux  Inputs=2
  Mux2 : Mux  Inputs=3
  Relational Operator : RelationalOperator  Operator=<  OutDataTypeStr=boolean  InputSameDT=off
  Scope : Scope
  Scope1 : Scope
  Scope2 : Scope
  Sign : Signum
  Switch : Switch  Criteria=u2 > Threshold  SaturateOnIntegerOverflow=off  InputSameDT=off
  Terminator : Terminator
  To Workspace : ToWorkspace  VariableName=crack_size  SaveFormat=Structure With Time  SampleTime=-1
  Transfer Fcn : TransferFcn  Denominator=[1/(2*pi*1000) 1]
  crack_size calculation : Subsystem
  Kw_mod : Outport
  wires:
  Memory3/1 -> Bending (normal) stress computation/2(Crack_size[mm])
  Derivative/1 -> Sign/1
  Mux/1 -> Enabled Subsystem/1(max,min)
  Bending (normal) stress computation/1(sigma [MPa]) -> MinMax Running Resettable/1, MinMax Running Resettable1/1, Abs/1
  MinMax Running Resettable/1 -> Mux/1
  MinMax Running Resettable1/1 -> Mux/2
  Enabled Subsystem/1(DeltaS_side1) -> Mux1/1
  Enabled Subsystem/2(DeltaS_side2) -> Mux1/2
  Mux1/1 -> crack_size calculation/1(Delta_S)
  crack_size calculation/1(crack_size [mm]) -> Scope1/1, To Workspace/1, Mux2/2
  Constant1/1 -> Mux2/1, Mux3/1
  Constant2/1 -> Relational Operator/2
  Relational Operator/1 -> Data Type Conversion/1
  Fcn/1 -> Kw_mod/1
  Sign/1 -> Detect Change/1
  Detect Change/1 -> Memory2/1, Enabled Subsystem/Enable, crack_size calculation/Enable
  Constant3/1 -> Switch/1
  Constant4/1 -> Add1/1
  Add/1 -> Memory1/1
  Memory1/1 -> Add2/2, Add/2
  Add1/1 -> Add/1
  Constant5/1 -> Switch/3
  Switch/1 -> Mux2/3, Add1/2
  Data Type Conversion/1 -> Add2/1
  Add2/1 -> Switch/2
  Fcn1/1 -> Mux3/2, Memory3/1
  Mux3/1 -> Fcn/1
  Memory2/1 -> MinMax Running Resettable1/2, MinMax Running Resettable/2
  Mux2/1 -> Fcn1/1
  Enabled Subsystem/3(Reset_minmax) -> Terminator/1
  Abs/1 -> Scope/1, Relational Operator/1
  Tb [N/m]/1 -> Mux4/1, Transfer Fcn/1
  Mux4/1 -> Scope2/1
  Transfer Fcn/1 -> Mux4/2, Derivative/1, Bending (normal) stress computation/1(Tb [Nm])

== system Modello_attuatore/Actuation System/Servovalve/Servovalve Dynamic/First Stage Leakage ==
  In1 : Inport
  In2 : Inport  Port=2
  In4 : Inport  Port=3
  Add1 : Sum  Inputs=+|-
  Fcn : Fcn  Expr=0.22*sqrt(log(1+u(2)))*Afl_sv*sqrt(u(1))
  Memory : Memory  InitialCondition=5.74e-6
  Mux1 : Mux  Inputs=2
  Mux2 : Mux  Inputs=2
  Reynold : Fcn  Expr=u(1)*(u(3)/Afl_sv)*dfl_sv/(u(2))
  Saturation : Saturate  UpperLimit=5000  LowerLimit=0
  Out1 : Outport
  wires:
  Saturation/1 -> Mux1/2  "Re"
  In1/1 -> Add1/1  "Ps[Pa]"
  Reynold/1 -> Saturation/1  "Re"
  Mux1/1 -> Fcn/1
  Fcn/1 -> Out1/1, Memory/1  "QLfs[m3/s]"
  Add1/1 -> Mux1/1  "dP[Pa]"
  In2/1 -> Add1/2  "Pr[Pa]"
  Mux2/1 -> Reynold/1
  In4/1 -> Mux2/1  "ro;mu"
  Memory/1 -> Mux2/2  "Qlfs[m3/s]"

== system Modello_attuatore/Actuation System/Servovalve/Servovalve Dynamic/Hydraulic amplifier ==
  In4 : Inport
  In2 : Inport  Port=2
  In3 : Inport  Port=3
  In1 : Inport  Port=4
  In5 : Inport  Port=5
  Add2 : Sum  Inputs=+|-
  Jetpipe area occlusion : Subsystem
  Scope3 : Scope
  Ugello A : Subsystem
  Ugello B : Subsystem
  Out1 : Outport
  wires:
  In1/1 -> Ugello A/2(In2), Ugello B/4(In2)  "dxs[m/s]"
  Add2/1 -> Out1/1  "Dp"
  Ugello B/1(PB) -> Add2/2
  Ugello A/1(PA) -> Add2/1
  In4/1 -> Ugello A/1(In4), Ugello B/5(In4)  "xf[m]"
  In2/1 -> Ugello A/3(In1), Ugello B/3(In1)
  In3/1 -> Ugello A/4(In3), Ugello B/2(In3)
  Jetpipe area occlusion/1(Out2) -> Ugello B/1(In5), Scope3/1, Ugello A/5(In5)
  In5/1 -> Jetpipe area occlusion/1(In1)

== system Modello_attuatore/Actuation System/Servovalve/Servovalve Dynamic/Jet pipe dynamic ==
  In1 : Inport
  In4 : Inport  Port=2
  In2 : Inport  Port=3
  Add1 : Sum  Inputs=+|-|-|-
  Add2 : Sum  Inputs=+|+
  Dead Zone : DeadZone  LowerValue=-gap_ms/2  UpperValue=gap_ms/2
  Double Integrator : Subsystem
  Gain : Gain  Gain=1/Ja_sv
  Gain1 : Gain  Gain=Kw_sv
  Gain3 : Gain  Gain=Kf_sv
  Gain4 : Gain  Gain=bf_sv
  Gain5 : Gain  Gain=0.7
  Jetpipe distorted : Subsystem
  Mux1 : Mux  Inputs=2
  Product1 : Product  SaturateOnIntegerOverflow=on  OutDataTypeStr=Inherit: Same as first input
  Scope : Scope
  Out1 : Outport
  Out2 : Outport  Port=2
  wires:
  In4/1 -> Add1/1  "Torque [N]"
  Add1/1 -> Gain/1
  Gain/1 -> Double Integrator/1(In1)  "ddxf[m2/s]"
  Jetpipe distorted/1(Out2) -> Add2/2, Gain3/1, Out1/1, Gain5/1, Mux1/2  "xf[m]"
  Gain3/1 -> Add1/3
  Gain5/1 -> Out2/1  "xa[m]"
  Add2/1 -> Dead Zone/1
  In1/1 -> Add2/1  "xs[m]"
  Gain4/1 -> Add1/4
  Double Integrator/2(Out2) -> Gain4/1
  Dead Zone/1 -> Gain1/1
  [turbolence_on_jetpipe] -> Jetpipe distorted/1(In3)
  Double Integrator/1(Out1) -> Jetpipe distorted/2(In1), Mux1/1
  Mux1/1 -> Scope/1
  Product1/1 -> Add1/2
  In2/1 -> Product1/1  "Kw_modifier"
  Gain1/1 -> Product1/2  "Fb[Nm]"

== system Modello_attuatore/Actuation System/Servovalve/Servovalve Dynamic/Spool  dynamic ==
  In1 : Inport
  In4 : Inport  Port=2
  In2 : Inport  Port=3
  Add1 : Sum  Inputs=-|+
  Add2 : Sum  Inputs=+|+
  Add3 : Sum  Inputs=+|+
  Dead Zone : DeadZone  LowerValue=-gap_ms/2  UpperValue=gap_ms/2
  Double Integrator : Subsystem
  Flow Force : Subsystem
  Friction : Subsystem
  Gain : Gain  Gain=1/msp_sv
  Gain2 : Gain  Gain=Kw_sv/lf
  Gain3 : Gain  Gain=Asp_sv
  Product1 : Product  SaturateOnIntegerOverflow=on  OutDataTypeStr=Inherit: Same as first input
  Out1 : Outport
  Out2 : Outport  Port=2
  wires:
  Gain/1 -> Double Integrator/1(In1)  "ddxs [m2/s]"
  Double Integrator/2(Out2) -> Out2/1, Friction/2(In2)  "dxs[m/s]"
  Double Integrator/1(Out1) -> Out1/1, Flow Force/1(In1), Add2/1  "xs[m]"
  In4/1 -> Gain3/1  "dP[Pa]"
  Gain3/1 -> Add1/2
  In1/1 -> Add2/2  "xf[m]"
  Add2/1 -> Dead Zone/1
  Friction/1(Out1) -> Gain/1
  Dead Zone/1 -> Gain2/1
  Add3/1 -> Friction/1(In1)  "F_res [N]"
  Add1/1 -> Add3/2  "F_res [N]"
  Friction/2(Out2) -> Double Integrator/2(In2)
  Double Integrator/3(Out3) -> Friction/3(In3)
  Flow Force/1(Ffl1+Ffl2) -> Add3/1
  Gain2/1 -> Product1/1  "Ffb[N]"
  In2/1 -> Product1/2  "Kw_modifier"
  Product1/1 -> Add1/1

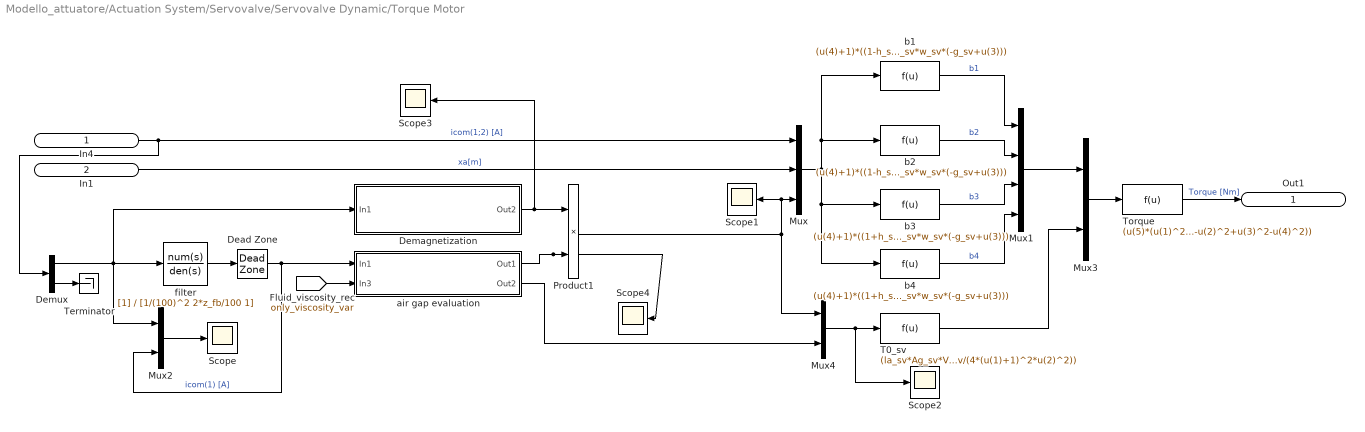
== system Modello_attuatore/Actuation System/Servovalve/Servovalve Dynamic/Torque Motor ==
  In4 : Inport
  In1 : Inport  Port=2
  Dead Zone : DeadZone  LowerValue=-0.025*imax_sv  UpperValue=0.025*imax_sv
  Demagnetization : Subsystem
  Demux : Demux  Outputs=2
  Mux : Mux  Inputs=3
  Mux1 : Mux
  Mux2 : Mux  Inputs=2
  Mux3 : Mux  Inputs=2
  Mux4 : Mux  Inputs=2
  Product1 : Product  SaturateOnIntegerOverflow=on  OutDataTypeStr=Inherit: Same as first input
  Scope{,1..4} (5 alike) : Scope
  T0_sv : Fcn  Expr=(la_sv*Ag_sv*Vp_sv^2*mua_sv/(4*(u(1)+1)^2*u(2)^2))
  Terminator : Terminator
  Torque : Fcn  Expr=(u(5)*(u(1)^2-u(2)^2+u(3)^2-u(4)^2))
  air gap evaluation : Subsystem
  b1 : Fcn  Expr=(u(4)+1)*((1-h_sv)*(1+h_sv+w_sv-g_sv+u(3))+(n1_sv*u(1)+n2_sv*u(2))/Vp_sv*((u(4)+1)*(1-h_sv)+(-g_sv+u(3))*(1+w_sv)-h_sv*w_sv-w_sv^2))/((u(4)+1)*(1-h_sv^2)-w_sv^2-(-g_sv+u(3))^2+2*h_sv*w_sv*(-g_sv+u(3)))
  b2 : Fcn  Expr=(u(4)+1)*((1-h_sv)*(1+h_sv-w_sv+g_sv-u(3))-(n1_sv*u(1)+n2_sv*u(2))/Vp_sv*((u(4)+1)*(1-h_sv)-(-g_sv+u(3))*(1-w_sv)+h_sv*w_sv-w_sv^2))/((u(4)+1)*(1-h_sv^2)-w_sv^2-(-g_sv+u(3))^2+2*h_sv*w_sv*(-g_sv+u(3)))
  b3 : Fcn  Expr=(u(4)+1)*((1+h_sv)*(1-h_sv-w_sv-g_sv+u(3))+(n1_sv*u(1)+n2_sv*u(2))/Vp_sv*((u(4)+1)*(1+h_sv)+(-g_sv+u(3))*(1-w_sv)-h_sv*w_sv-w_sv^2))/((u(4)+1)*(1-h_sv^2)-w_sv^2-(-g_sv+u(3))^2+2*h_sv*w_sv*(-g_sv+u(3)))
  b4 : Fcn  Expr=(u(4)+1)*((1+h_sv)*(1-h_sv+w_sv+g_sv-u(3))-(n1_sv*u(1)+n2_sv*u(2))/Vp_sv*((u(4)+1)*(1+h_sv)-(-g_sv+u(3))*(1+w_sv)+h_sv*w_sv-w_sv^2))/((u(4)+1)*(1-h_sv^2)-w_sv^2-(-g_sv+u(3))^2+2*h_sv*w_sv*(-g_sv+u(3)))
  filter : TransferFcn  Denominator=[1/(100)^2 2*z_fb/100 1]
  Out1 : Outport
  wires:
  Mux/1 -> b2/1, b1/1, b3/1, b4/1
  In1/1 -> Mux/2  "xa[m]"
  In4/1 -> Mux/1, Demux/1  "icom(1;2) [A]"
  Torque/1 -> Out1/1  "Torque [Nm]"
  b3/1 -> Mux1/3  "b3"
  b4/1 -> Mux1/4  "b4"
  b2/1 -> Mux1/2  "b2"
  b1/1 -> Mux1/1  "b1"
  Mux2/1 -> Scope/1
  filter/1 -> Dead Zone/1
  Demux/2 -> Terminator/1
  Demux/1 -> filter/1, Mux2/1, Demagnetization/1(In1)
  Dead Zone/1 -> Mux2/2, air gap evaluation/1(In1)  "icom(1) [A]"
  Product1/1 -> Mux/3, Scope1/1, Mux4/1
  Mux3/1 -> Torque/1
  Mux1/1 -> Mux3/1
  T0_sv/1 -> Mux3/2
  [only_viscosity_var] -> air gap evaluation/2(In3)
  Mux4/1 -> T0_sv/1, Scope2/1
  air gap evaluation/2(Out2) -> Mux4/2
  air gap evaluation/1(Out1) -> Product1/2, Scope4/1
  Demagnetization/1(Out2) -> Product1/1, Scope3/1

== system Modello_attuatore/Actuation System/Servovalve/Spool/orifice1R-flow ==
  In4 : Inport
  In1 : Inport  Port=2
  In2 : Inport  Port=3
  Gain : Gain  Gain=4  SaturateOnIntegerOverflow=on  OutDataTypeStr=Inherit: Same as input  ParamDataTypeStr=Inherit: Same as input
  Gain1 : Gain  Gain=2  SaturateOnIntegerOverflow=on  OutDataTypeStr=Inherit: Same as input  ParamDataTypeStr=Inherit: Same as input
  Math Function : Math  Operator=sqrt  SignedPower=on
  Math Function1 : Math  Operator=magnitude^2  SignedPower=on
  Product : Product  Inputs=3  SaturateOnIntegerOverflow=on  OutDataTypeStr=Inherit: Same as first input
  Product1 : Product  Inputs=*/  SaturateOnIntegerOverflow=on  OutDataTypeStr=Inherit: Same as first input
  Product2 : Product  SaturateOnIntegerOverflow=on  OutDataTypeStr=Inherit: Same as first input
  Sign : Signum
  Sum : Sum  Inputs=|++  SaturateOnIntegerOverflow=on
  Sum1 : Sum  Inputs=|+-  SaturateOnIntegerOverflow=on
  Out4 : Outport
  wires:
  Product2/1 -> Out4/1  "Q_1R[m3/s]"
  In2/1 -> Math Function1/1, Sum1/2  "R_CR1"
  Product1/1 -> Product2/2
  Gain1/1 -> Product1/2
  Sum1/1 -> Product1/1
  Math Function/1 -> Sum1/1
  Sum/1 -> Math Function/1
  Math Function1/1 -> Sum/2
  Gain/1 -> Sum/1
  Product/1 -> Gain/1
  In1/1 -> Product/3, Gain1/1  "R_AR1"
  In4/1 -> Product/2, Sign/1  "dP[Pa]"
  Sign/1 -> Product2/1, Product/1

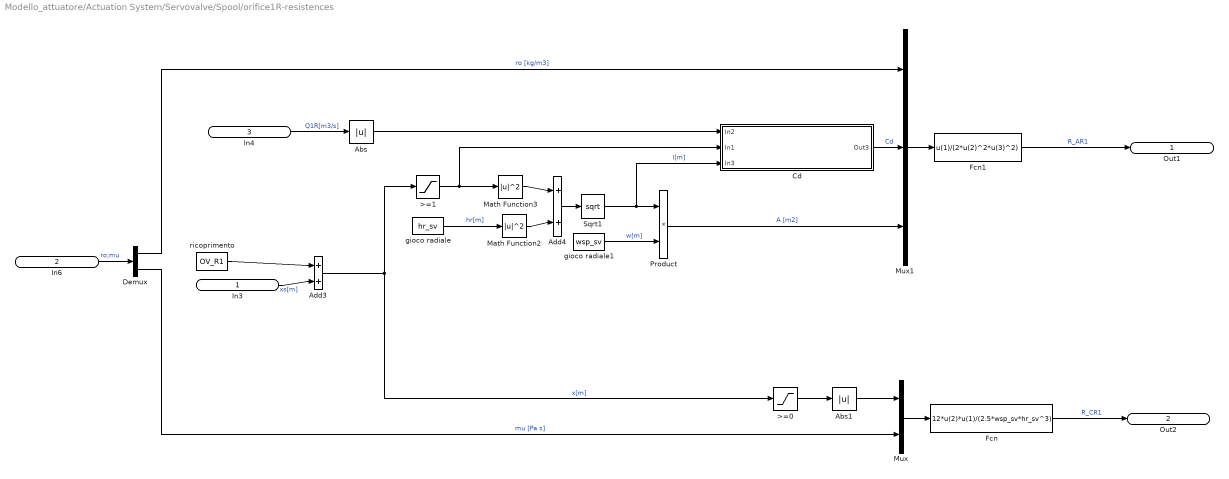
== system Modello_attuatore/Actuation System/Servovalve/Spool/orifice1R-resistences ==
  In3 : Inport
  In6 : Inport  Port=2
  In4 : Inport  Port=3
  >=0 : Saturate  UpperLimit=inf  LowerLimit=0
  >=1 : Saturate  UpperLimit=0  LowerLimit=-inf
  Abs : Abs  SaturateOnIntegerOverflow=off
  Abs1 : Abs  SaturateOnIntegerOverflow=off
  Add3 : Sum  Inputs=+|+
  Add4 : Sum  Inputs=+|+
  Cd : Subsystem
  Demux : Demux  Outputs=2
  Fcn : Fcn  Expr=12*u(2)*u(1)/(2.5*wsp_sv*hr_sv^3)
  Fcn1 : Fcn  Expr=u(1)/(2*u(2)^2*u(3)^2)
  Math Function2 : Math  Operator=magnitude^2  SignedPower=on
  Math Function3 : Math  Operator=magnitude^2  SignedPower=on
  Mux : Mux  Inputs=2
  Mux1 : Mux  Inputs=3
  Product : Product  RndMeth=Zero
  Sqrt1 : Sqrt  AlgorithmType=Newton-Raphson
  gioco radiale : Constant  Value=hr_sv
  gioco radiale1 : Constant  Value=wsp_sv
  ricoprimento : Constant  Value=OV_R1
  Out1 : Outport
  Out2 : Outport  Port=2
  wires:
  Mux/1 -> Fcn/1
  Mux1/1 -> Fcn1/1
  Fcn1/1 -> Out1/1  "R_AR1"
  Demux/2 -> Mux/2  "mu [Pa s]"
  Cd/1(Out3) -> Mux1/2  "Cd"
  In4/1 -> Abs/1  "Q1R[m3/s]"
  Demux/1 -> Mux1/1  "ro [kg/m3]"
  In6/1 -> Demux/1  "ro;mu"
  ricoprimento/1 -> Add3/1
  In3/1 -> Add3/2  "xs[m]"
  Abs/1 -> Cd/1(In2)
  gioco radiale/1 -> Math Function2/1  "hr[m]"
  Add3/1 -> >=1/1, >=0/1  "x[m]"
  >=0/1 -> Abs1/1
  Add4/1 -> Sqrt1/1
  Math Function3/1 -> Add4/1
  Math Function2/1 -> Add4/2
  gioco radiale1/1 -> Product/2  "w[m]"
  Abs1/1 -> Mux/1
  >=1/1 -> Math Function3/1, Cd/2(In1)
  Sqrt1/1 -> Product/1, Cd/3(In3)  "l[m]"
  Product/1 -> Mux1/3  "A [m2]"
  Fcn/1 -> Out2/1  "R_CR1"

== system Modello_attuatore/Actuation System/Servovalve/Spool/orifice1S-resistences ==
  In3 : Inport
  In6 : Inport  Port=2
  In4 : Inport  Port=3
  >=0 : Saturate  UpperLimit=0  LowerLimit=-inf
  >=1 : Saturate  UpperLimit=inf  LowerLimit=0
  Abs : Abs  SaturateOnIntegerOverflow=off
  Abs1 : Abs  SaturateOnIntegerOverflow=off
  Add3 : Sum  Inputs=-|+
  Add4 : Sum  Inputs=+|+
  Cd : Subsystem
  Demux : Demux  Outputs=2
  Fcn : Fcn  Expr=12*u(2)*u(1)/(2.5*wsp_sv*hr_sv^3)
  Fcn1 : Fcn  Expr=u(1)/(2*u(2)^2*u(3)^2)
  Math Function2 : Math  Operator=magnitude^2  SignedPower=on
  Math Function3 : Math  Operator=magnitude^2  SignedPower=on
  Mux : Mux  Inputs=2
  Mux1 : Mux  Inputs=3
  Product : Product  RndMeth=Zero
  Sqrt1 : Sqrt  AlgorithmType=Newton-Raphson
  gioco radiale : Constant  Value=hr_sv
  gioco radiale1 : Constant  Value=wsp_sv
  ricoprimento : Constant  Value=OV_S1
  Out1 : Outport
  Out2 : Outport  Port=2
  wires:
  Mux/1 -> Fcn/1
  Mux1/1 -> Fcn1/1
  Fcn1/1 -> Out1/1  "R_AS1"
  Demux/2 -> Mux/2  "mu [Pa s]"
  Cd/1(Out3) -> Mux1/2  "Cd"
  In4/1 -> Abs/1  "Q1S[m3/s]"
  Demux/1 -> Mux1/1  "ro [kg/m3]"
  In6/1 -> Demux/1  "ro;mu"
  ricoprimento/1 -> Add3/1
  In3/1 -> Add3/2  "xs[m]"
  Abs/1 -> Cd/1(In2)
  gioco radiale/1 -> Math Function2/1  "hr[m]"
  Add3/1 -> >=1/1, >=0/1  "x[m]"
  >=0/1 -> Abs1/1
  Add4/1 -> Sqrt1/1
  Math Function3/1 -> Add4/1
  Math Function2/1 -> Add4/2
  gioco radiale1/1 -> Product/2  "w[m]"
  Abs1/1 -> Mux/1
  >=1/1 -> Math Function3/1, Cd/2(In1)
  Sqrt1/1 -> Product/1, Cd/3(In3)  "l[m]"
  Product/1 -> Mux1/3  "A [m2]"
  Fcn/1 -> Out2/1  "R_CS1"

== system Modello_attuatore/Actuation System/Servovalve/Spool/orifice2R-flow ==
  In4 : Inport
  In1 : Inport  Port=2
  In2 : Inport  Port=3
  Gain : Gain  Gain=4  SaturateOnIntegerOverflow=on  OutDataTypeStr=Inherit: Same as input  ParamDataTypeStr=Inherit: Same as input
  Gain1 : Gain  Gain=2  SaturateOnIntegerOverflow=on  OutDataTypeStr=Inherit: Same as input  ParamDataTypeStr=Inherit: Same as input
  Math Function : Math  Operator=sqrt  SignedPower=on
  Math Function1 : Math  Operator=magnitude^2  SignedPower=on
  Product : Product  Inputs=3  SaturateOnIntegerOverflow=on  OutDataTypeStr=Inherit: Same as first input
  Product1 : Product  Inputs=*/  SaturateOnIntegerOverflow=on  OutDataTypeStr=Inherit: Same as first input
  Product2 : Product  SaturateOnIntegerOverflow=on  OutDataTypeStr=Inherit: Same as first input
  Sign : Signum
  Sum : Sum  Inputs=|++  SaturateOnIntegerOverflow=on
  Sum1 : Sum  Inputs=|+-  SaturateOnIntegerOverflow=on
  Out4 : Outport
  wires:
  Sign/1 -> Product/1, Product2/1
  In4/1 -> Product/2, Sign/1  "dP[Pa]"
  In1/1 -> Gain1/1, Product/3  "R_AR2"
  Product/1 -> Gain/1
  Gain/1 -> Sum/1
  Math Function1/1 -> Sum/2
  Sum/1 -> Math Function/1
  Math Function/1 -> Sum1/1
  Sum1/1 -> Product1/1
  Gain1/1 -> Product1/2
  Product1/1 -> Product2/2
  In2/1 -> Sum1/2, Math Function1/1  "R_CR2"
  Product2/1 -> Out4/1  "Q_2R[m3/s]"
